simulink model "ciagly_zlinearyzowany_model_dynamiczny"  (R2022b)
settings: Solver=VariableStepAuto  StartTime=0.0  StopTime=100  RelTol=1e-3
values from neighbouring files (symbols this model uses):
  a0 = 0.00185185    [Projekt1.m]    (also in transmitancja_dyskretna.m = data.a0; wykresy_char_stat_nlin.m = data.a0; wykresy_char_stat_zlin.m = data.a0)
  a1 = 0.0462963    [Projekt1.m]    (also in transmitancja_dyskretna.m = data.a1; wykresy_char_stat_nlin.m = data.a1; wykresy_char_stat_zlin.m = data.a1)
  a2 = 0.377778    [Projekt1.m]    (also in transmitancja_dyskretna.m = data.a2; wykresy_char_stat_nlin.m = data.a2; wykresy_char_stat_zlin.m = data.a2)
  alpha1 = 0.4    [Projekt1.m]    (also in transmitancja_dyskretna.m = data.alpha1; wykresy_char_stat_nlin.m = data.alpha1; wykresy_char_stat_zlin.m = data.alpha1)
  alpha2 = 0.55    [Projekt1.m]    (also in transmitancja_dyskretna.m = data.alpha2; wykresy_char_stat_nlin.m = data.alpha2; wykresy_char_stat_zlin.m = data.alpha2)
  alpha3 = -0.92    [Projekt1.m]    (also in transmitancja_dyskretna.m = data.alpha3; wykresy_char_stat_nlin.m = data.alpha3; wykresy_char_stat_zlin.m = data.alpha3)
  alpha4 = 0.53    [Projekt1.m]    (also in transmitancja_dyskretna.m = data.alpha4; wykresy_char_stat_nlin.m = data.alpha4; wykresy_char_stat_zlin.m = data.alpha4)
  b0 = 0.00333333    [Projekt1.m]    (also in transmitancja_dyskretna.m = data.b0; wykresy_char_stat_nlin.m = data.b0; wykresy_char_stat_zlin.m = data.b0)
  t_u_step_sim = 1    [Projekt1.m]    (also in wykresy_char_dyn_dys.m)
  u_step_sim = 1    [Projekt1.m]    (also in wykresy_char_dyn_dys.m)
  ud = uds(i)    [Projekt1.m]
  X_0 = [0;0;0]    [Projekt1.m]
settings Model: Creator=pioro  LastModifiedBy=pioro

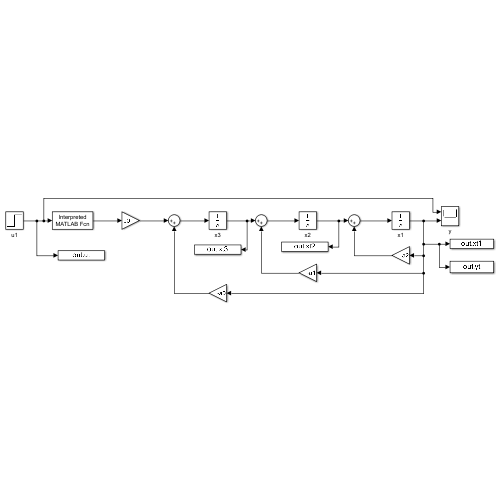
[thumbnail: Simulink's stored preview of the top-level diagram]
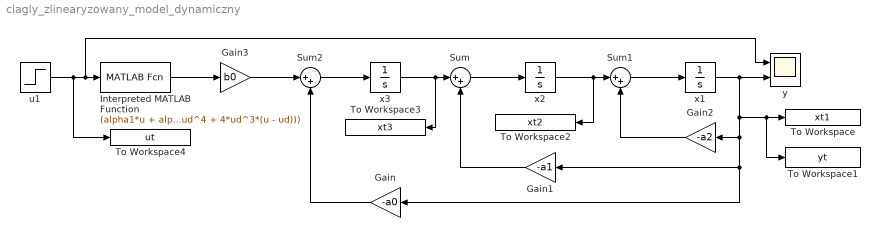
== system ciagly_zlinearyzowany_model_dynamiczny ==
  Gain : Gain  Gain=-a0
  Gain1 : Gain  Gain=-a1
  Gain2 : Gain  Gain=-a2
  Gain3 : Gain  Gain=b0
  Interpreted MATLAB Function : MATLABFcn  MATLABFcn=(alpha1*u + alpha2*(2*ud*(u - ud) + ud^2) + alpha3*(ud^3 + 3*ud^2*(u - ud)) + alpha4*(ud^4 + 4*ud^3*(u - ud)))
  Sum : Sum  Inputs=|++
  Sum1 : Sum  Inputs=|++
  Sum2 : Sum  Inputs=|++
  To Workspace : ToWorkspace  VariableName=xt1  SaveFormat=Timeseries  SampleTime=-1
  To Workspace1 : ToWorkspace  VariableName=yt  SaveFormat=Timeseries  SampleTime=-1
  To Workspace2 : ToWorkspace  VariableName=xt2  SaveFormat=Timeseries  SampleTime=-1
  To Workspace3 : ToWorkspace  VariableName=xt3  SaveFormat=Timeseries  SampleTime=-1
  To Workspace4 : ToWorkspace  VariableName=ut  SaveFormat=Timeseries  SampleTime=-1
  u1 : Step  Time=t_u_step_sim  After=u_step_sim  SampleTime=0
  x1 : Integrator  InitialCondition=X_0(1)
  x2 : Integrator  InitialCondition=X_0(2)
  x3 : Integrator  InitialCondition=X_0(3)
  y : Scope  NumInputPorts=2
  wires:
  x3/1 -> To Workspace3/1, Sum/1
  x2/1 -> To Workspace2/1, Sum1/1
  Sum/1 -> x2/1
  Gain/1 -> Sum2/2
  Sum1/1 -> x1/1
  Gain3/1 -> Sum2/1
  Gain1/1 -> Sum/2
  Gain2/1 -> Sum1/2
  Interpreted MATLAB Function/1 -> Gain3/1
  Sum2/1 -> x3/1
  u1/1 -> To Workspace4/1, y/1, Interpreted MATLAB Function/1
  x1/1 -> To Workspace1/1, To Workspace/1, Gain/1, Gain1/1, Gain2/1, y/2
